simulink model "sampleModel7127_pp_difftest"  (R2018a)
settings: Solver=VariableStepAuto  StartTime=0.0  StopTime=10.0  RelTol=1e-3
undefined symbols (not defined in the file or in its folder): DiscIntNeverNeededParam, sigbuilder_block
libraries: simulink x258
(part 1 of 5)
settings Model: Creator=cyfuzz  LastModifiedBy=ishaf
settings CodeAppCC: StateflowObjectComments=on

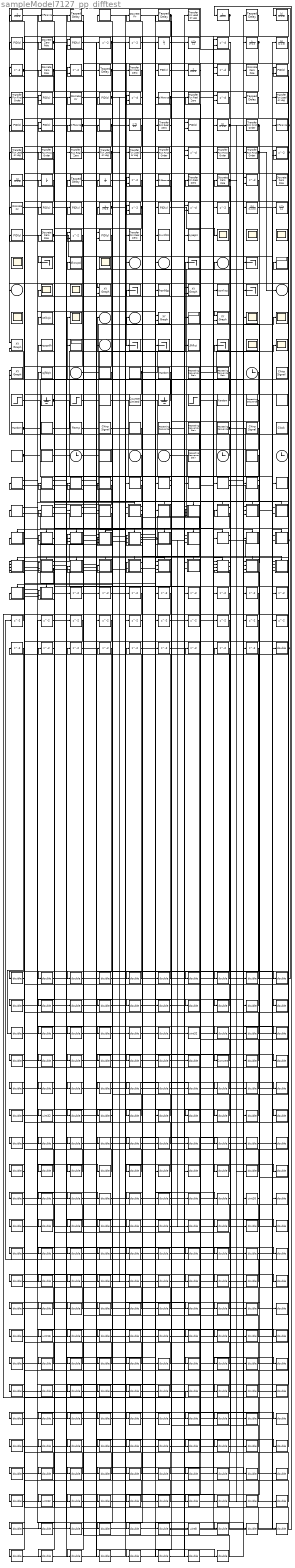
== system sampleModel7127_pp_difftest ==
  cfblk133 : Inport
  cfblk165 : Inport  Port=2
  cfblk166 : Inport  Port=3
  cfblk{1,8,19,27,74} (5 alike) : DiscreteTransferFcn  SampleTime=1
  cfblk{10,20,48,61,79} (5 alike) : DiscreteFilter  SampleTime=1
  cfblk100 : Display
  cfblk{88..91,94,102..103,111,113,119..120,129..130} (13 alike) : Scope
      cfblk103 settings: Floating=on
      cfblk111 settings: Floating=on
      cfblk129 settings: Floating=on
      cfblk89 settings: Floating=on
      cfblk90 settings: Floating=on
      cfblk91 settings: Floating=on
      cfblk94 settings: Floating=on
  cfblk{104,107,116,118,121,131} (6 alike) : simulink/Sinks/XY Graph  xmin=-1  xmax=1  ymin=-1  ymax=1  st=-1
  cfblk{92,97,99,105,109,125..126,128} (8 alike) : Terminator
  cfblk106 : ToWorkspace  VariableName=hqnbljg  SaveFormat=Timeseries  SampleTime=-1
  cfblk108 : ToWorkspace  VariableName=kqrxkcy  SaveFormat=Timeseries  SampleTime=-1
  cfblk{11,26,34,41,72..73,76,81} (8 alike) : simulink/Continuous/PID Controller  Controller=PID  TimeDomain=Discrete-time  SampleTime=1  IntegratorMethod=Forward Euler  FilterMethod=Forward Euler  Form=Parallel  UseFilter=on  ControllerParametersSource=internal  P=1  I=1  D=0  N=100  InitialConditionSource=internal  InitialConditionForIntegrator=0  InitialConditionForFilter=0  ExternalReset=none  LimitOutput=off  UpperSaturationLimit=inf  LowerSaturationLimit=-inf  LinearizeAsGain=off  AntiWindupMode=none  Kb=1  TrackingMode=off  Kt=1  PParamMin=[]  PParamMax=[]  IParamMin=[]  IParamMax=[]  DParamMin=[]  DParamMax=[]  NParamMin=[]  NParamMax=[]  KbParamMin=[]  KbParamMax=[]  KtParamMin=[]  KtParamMax=[]  POutMin=[]  POutMax=[]  IOutMin=[]  IOutMax=[]  DOutMin=[]  DOutMax=[]  NOutMin=[]  NOutMax=[]  KbOutMin=[]  KbOutMax=[]  KtOutMin=[]  KtOutMax=[]  IntegratorOutMin=[]  IntegratorOutMax=[]  FilterOutMin=[]  FilterOutMax=[]  SumOutMin=[]  SumOutMax=[]  SumI1OutMin=[]  SumI1OutMax=[]  SumI2OutMin=[]  SumI2OutMax=[]  SumI3OutMin=[]  SumI3OutMax=[]  SumDOutMin=[]  SumDOutMax=[]  SaturationOutMin=[]  SaturationOutMax=[]  IntegratorContinuousStateAttributes=''  IntegratorStateMustResolveToSignalObject=off  IntegratorRTWStateStorageClass=Auto  FilterContinuousStateAttributes=''  FilterStateMustResolveToSignalObject=off  FilterRTWStateStorageClass=Auto  DifferentiatorICPrevScaledInput=0  DifferentiatorOutMin=[]  DifferentiatorOutMax=[]  FilterDiffOutCoefMin=[]  FilterDiffOutCoefMax=[]  SumDenOutMin=[]  SumDenOutMax=[]  SumNumOutMin=[]  SumNumOutMax=[]  ReciprocalOutMin=[]  ReciprocalOutMax=[]  DivideOutMin=[]  DivideOutMax=[]  TunerSelectOption=Transfer Function Based (PID Tuner App)
  cfblk112 : ToWorkspace  VariableName=otikzjx  SaveFormat=Timeseries  SampleTime=-1
  cfblk117 : Display
  cfblk{12,22,29,68,70,82} (6 alike) : DiscreteZeroPole  Poles=[0 0.5]  Gain=1
  cfblk122 : ToWorkspace  VariableName=rqzqsdh  SaveFormat=Timeseries  SampleTime=-1
  cfblk123 : Display
  cfblk127 : ToWorkspace  VariableName=jlhlkzi  SaveFormat=Timeseries  SampleTime=-1
  cfblk{13,30,32,42,47,84} (6 alike) : simulink/Continuous/PID Controller (2DOF)  Controller=PID  TimeDomain=Discrete-time  SampleTime=1  IntegratorMethod=Forward Euler  FilterMethod=Forward Euler  Form=Parallel  UseFilter=on  ControllerParametersSource=internal  P=1  I=1  D=0  N=100  b=1  c=1  InitialConditionSource=internal  InitialConditionForIntegrator=0  InitialConditionForFilter=0  ExternalReset=none  LimitOutput=off  UpperSaturationLimit=inf  LowerSaturationLimit=-inf  LinearizeAsGain=off  AntiWindupMode=none  Kb=1  TrackingMode=off  Kt=1  PParamMin=[]  PParamMax=[]  IParamMin=[]  IParamMax=[]  DParamMin=[]  DParamMax=[]  NParamMin=[]  NParamMax=[]  bParamMin=[]  bParamMax=[]  cParamMin=[]  cParamMax=[]  KbParamMin=[]  KbParamMax=[]  KtParamMin=[]  KtParamMax=[]  POutMin=[]  POutMax=[]  IOutMin=[]  IOutMax=[]  DOutMin=[]  DOutMax=[]  NOutMin=[]  NOutMax=[]  bOutMin=[]  bOutMax=[]  cOutMin=[]  cOutMax=[]  KbOutMin=[]  KbOutMax=[]  KtOutMin=[]  KtOutMax=[]  IntegratorOutMin=[]  IntegratorOutMax=[]  FilterOutMin=[]  FilterOutMax=[]  SumOutMin=[]  SumOutMax=[]  Sum1OutMin=[]  Sum1OutMax=[]  Sum2OutMin=[]  Sum2OutMax=[]  Sum3OutMin=[]  Sum3OutMax=[]  SumI1OutMin=[]  SumI1OutMax=[]  SumI2OutMin=[]  SumI2OutMax=[]  SumI3OutMin=[]  SumI3OutMax=[]  SumDOutMin=[]  SumDOutMax=[]  SaturationOutMin=[]  SaturationOutMax=[]  IntegratorContinuousStateAttributes=''  IntegratorStateMustResolveToSignalObject=off  IntegratorRTWStateStorageClass=Auto  FilterContinuousStateAttributes=''  FilterStateMustResolveToSignalObject=off  FilterRTWStateStorageClass=Auto  DifferentiatorICPrevScaledInput=0  DifferentiatorOutMin=[]  DifferentiatorOutMax=[]  FilterDiffOutCoefMin=[]  FilterDiffOutCoefMax=[]  SumDenOutMin=[]  SumDenOutMax=[]  SumNumOutMin=[]  SumNumOutMax=[]  ReciprocalOutMin=[]  ReciprocalOutMax=[]  DivideOutMin=[]  DivideOutMax=[]  TunerSelectOption=Transfer Function Based (PID Tuner App)
  cfblk132 : ToWorkspace  VariableName=qjfdqit  SaveFormat=Timeseries  SampleTime=-1
  cfblk{134..135,161,169} (4 alike) : simulink/Sources/Band-Limited White Noise  Cov=[0.1]  Ts=0.1  seed=[23341]
  cfblk136 : RandomNumber  SampleTime=0.1
  cfblk{137..138,157,167} (4 alike) : simulink/Sources/Repeating Sequence Stair  OutValues=[3 1 4 2 1].'  tsamp=1  OutMin=[]  OutMax=[]  OutDataTypeStr=double  OutputDataTypeScalingMode=double  OutDataType=fixdt(0,8)  ConRadixGroup=Best Precision: Vector-wise  OutScaling=2^-12
  cfblk{139,163,168,170} (4 alike) : Clock
  cfblk{14..15,78,213..239} (30 alike) : Delay  SampleTime=1
  cfblk140 : simulink/Sources/Chirp Signal  f1=0.1  T=100  f2=1
  cfblk141 : Step  After=53  SampleTime=0
  cfblk142 : Ground
  cfblk143 : Step  After=78  SampleTime=0
  cfblk144 : simulink/Sources/Counter Free-Running  NumBits=16  tsamp=1
  cfblk145 : simulink/Sources/Counter Limited  uplimit=7  tsamp=1
  cfblk146 : Ground
  cfblk147 : Step  After=42  SampleTime=0
  cfblk148 : RandomNumber  SampleTime=0.1
  cfblk149 : simulink/Sources/Repeating Sequence  rep_seq_t=[0 2]  rep_seq_y=[0 2]
  cfblk150 : simulink/Sources/Repeating Sequence Interpolated  OutValues=[3 1 4 2 1].'  TimeValues=[0 0.1 0.5 0.6 1].'  LookUpMeth=Interpolation-Use End Values  tsamp=0.01  OutMin=[]  OutMax=[]  OutDataTypeStr=double  OutputDataTypeScalingMode=double  OutDataType=fixdt(0,8)  OutScaling=2^-10
  cfblk151 : UniformRandomNumber  SampleTime=0.1
  cfblk152 : simulink/Sources/Repeating Sequence Interpolated  OutValues=[3 1 4 2 1].'  TimeValues=[0 0.1 0.5 0.6 1].'  LookUpMeth=Interpolation-Use End Values  tsamp=0.01  OutMin=[]  OutMax=[]  OutDataTypeStr=double  OutputDataTypeScalingMode=double  OutDataType=fixdt(0,8)  OutScaling=2^-10
  cfblk153 : simulink/Sources/Ramp  slope=1  start=0  InitialOutput=0
  cfblk154 : simulink/Sources/Chirp Signal  f1=0.1  T=100  f2=1
  cfblk155 : simulink/Sources/Counter Free-Running  NumBits=16  tsamp=1
  cfblk156 : simulink/Sources/Repeating Sequence  rep_seq_t=[0 2]  rep_seq_y=[0 2]
  cfblk158 : simulink/Sources/Repeating Sequence  rep_seq_t=[0 2]  rep_seq_y=[0 2]
  cfblk159 : simulink/Sources/Chirp Signal  f1=0.1  T=100  f2=1
  cfblk16 : UnitDelay
  cfblk160 : DigitalClock
  cfblk162 : Subsystem  Tag=STV Subsys  LoadFcn=sigbuilder_block('load');  StartFcn=sigbuilder_block('start');  StopFcn=sigbuilder_block('stop');  ClipboardFcn=sigbuilder_block('clipboard');  mask(Sigbuilder block){tuvar=[0:10]}
      mask help: Simulink:masks:SigbuilderBlock_MD
      mask init:
      | if ~strcmp(get_param(bdroot(gcbh),'SimulationStatus'),'stopped') tuvar = sigbuilder_block('maskInit'); end
      settings: CopyFcn=sigbuilder_block('copy');  DeleteFcn=sigbuilder_block('delete');  ModelCloseFcn=sigbuilder_block('modelClose');  PreSaveFcn=sigbuilder_block('preSave');  PauseFcn=sigbuilder_block('pause');  ContinueFcn=sigbuilder_block('continue');  NameChangeFcn=sigbuilder_block('namechange');  OpenFcn=sigbuilder_block('open',[437.6 199.2 550.4 400 ]);  CloseFcn=sigbuilder_block('close');
      mask Display: plot(0, 0, 100, 100,[2, 2, 32, 32, 2], [68, 8, 8, 68, 68],[32, 2], [38, 38], [32, 19, 2],[53, 60, 44], [32, 17, 17, 2],[16, 16, 31, 31]);txt = getActiveGroup(gcbh);text(2, 100, txt,'verticalAlignment', 'top');
  cfblk164 : Subsystem  Tag=STV Subsys  LoadFcn=sigbuilder_block('load');  StartFcn=sigbuilder_block('start');  StopFcn=sigbuilder_block('stop');  ClipboardFcn=sigbuilder_block('clipboard');  mask(Sigbuilder block){tuvar=[0:10]}
      mask help: Simulink:masks:SigbuilderBlock_MD
      mask init:
      | if ~strcmp(get_param(bdroot(gcbh),'SimulationStatus'),'stopped') tuvar = sigbuilder_block('maskInit'); end
      settings: CopyFcn=sigbuilder_block('copy');  DeleteFcn=sigbuilder_block('delete');  ModelCloseFcn=sigbuilder_block('modelClose');  PreSaveFcn=sigbuilder_block('preSave');  PauseFcn=sigbuilder_block('pause');  ContinueFcn=sigbuilder_block('continue');  NameChangeFcn=sigbuilder_block('namechange');  OpenFcn=sigbuilder_block('open',[437.6 199.2 550.4 400 ]);  CloseFcn=sigbuilder_block('close');
      mask Display: plot(0, 0, 100, 100,[2, 2, 32, 32, 2], [68, 8, 8, 68, 68],[32, 2], [38, 38], [32, 19, 2],[53, 60, 44], [32, 17, 17, 2],[16, 16, 31, 31]);txt = getActiveGroup(gcbh);text(2, 100, txt,'verticalAlignment', 'top');
  cfblk17 : DiscreteIntegrator  OutDataTypeStr=double  ICPrevOutput=DiscIntNeverNeededParam  ICPrevScaledInput=DiscIntNeverNeededParam
  cfblk{171..184} (14 alike) : If  SampleTime=1
  cfblk{18,28,35,38,57,69,77} (7 alike) : Delay  DelayLengthSource=Input port  SampleTime=1
      settings: InputPortMap=u0,p1
  cfblk185 : Subsystem  TreatAsAtomicUnit=on
  cfblk186 : Subsystem  TreatAsAtomicUnit=on
  cfblk187 : Subsystem  TreatAsAtomicUnit=on
  cfblk188 : Subsystem  TreatAsAtomicUnit=on
  cfblk189 : Subsystem  TreatAsAtomicUnit=on
  cfblk190 : Subsystem  TreatAsAtomicUnit=on
  cfblk191 : Subsystem  TreatAsAtomicUnit=on
  cfblk192 : Subsystem  TreatAsAtomicUnit=on
  cfblk193 : Subsystem  TreatAsAtomicUnit=on
  cfblk194 : Subsystem  TreatAsAtomicUnit=on
  cfblk195 : Subsystem  TreatAsAtomicUnit=on
  cfblk196 : Subsystem  TreatAsAtomicUnit=on
  cfblk197 : Subsystem  TreatAsAtomicUnit=on
  cfblk198 : Subsystem  TreatAsAtomicUnit=on
  cfblk199 : Subsystem  TreatAsAtomicUnit=on
  cfblk{2,36,43,50,66} (5 alike) : simulink/Discrete/Difference  ICPrevInput=0.0  OutMin=[]  OutMax=[]  OutDataTypeStr=double  OutputDataTypeScalingMode=double  OutDataType=fixdt(1, 16)  OutScaling=2^-10  DoSatur=off
  cfblk200 : Subsystem  TreatAsAtomicUnit=on
  cfblk201 : Subsystem  TreatAsAtomicUnit=on
  cfblk202 : Subsystem  TreatAsAtomicUnit=on
  cfblk203 : Subsystem  TreatAsAtomicUnit=on
  cfblk204 : Subsystem  TreatAsAtomicUnit=on
  cfblk205 : Subsystem  TreatAsAtomicUnit=on
  cfblk206 : Subsystem  TreatAsAtomicUnit=on
  cfblk207 : Subsystem  TreatAsAtomicUnit=on
  cfblk208 : Subsystem  TreatAsAtomicUnit=on
  cfblk209 : Subsystem  TreatAsAtomicUnit=on
  cfblk{21,23,60,65,75,83} (6 alike) : Delay  ShowEnablePort=on  SampleTime=1
      settings: InputPortMap=u0,e6
  cfblk210 : Subsystem  TreatAsAtomicUnit=on
  cfblk211 : Subsystem  TreatAsAtomicUnit=on
  cfblk212 : Subsystem  TreatAsAtomicUnit=on
  cfblk{3,6,9,24,39,63} (6 alike) : simulink/Discrete/Tapped Delay  vinit=0.0  samptime=-1  NumDelays=1  DelayOrder=Oldest  includeCurrent=off
  cfblk240 : DataTypeConversion  OutDataTypeStr=double
  cfblk{25,37,46,53,67,85} (6 alike) : simulink/Discrete/Transfer Fcn Real Zero  ZeroZ=0.75  ICPrevInput=0.0  DoSatur=off
      settings: SourceProductName=Simulink  SourceProductBaseCode=SL
  cfblk{31,49,52,56,58..59} (6 alike) : simulink/Discrete/Transfer Fcn First Order  PoleZ=0.95  ICPrevOutput=0.0  DoSatur=off
      settings: SourceProductName=Simulink
  cfblk33 : DiscreteFir  SampleTime=1
  cfblk4 : DiscreteStateSpace
  cfblk{7,40,51,54..55} (5 alike) : simulink/Discrete/Transfer Fcn Lead or Lag  PoleZ=0.95  ZeroZ=0.75  ICPrevOutput=0.0  ICPrevInput=0.0  DoSatur=off
      settings: SourceProductName=Simulink  SourceProductBaseCode=SL
  cfblk44 : DiscreteStateSpace
  cfblk45 : DiscreteIntegrator  OutDataTypeStr=double  ICPrevOutput=DiscIntNeverNeededParam  ICPrevScaledInput=DiscIntNeverNeededParam
  cfblk5 : DiscreteFir  SampleTime=1
  cfblk62 : UnitDelay
  cfblk64 : UnitDelay
  cfblk71 : DiscreteFir  SampleTime=1
  cfblk80 : DiscreteIntegrator  OutDataTypeStr=uint8  ICPrevOutput=DiscIntNeverNeededParam  ICPrevScaledInput=DiscIntNeverNeededParam
  cfblk86 : ToWorkspace  VariableName=zvvzltm  SaveFormat=Timeseries  SampleTime=-1
  cfblk87 : ToWorkspace  VariableName=sypegzn  SaveFormat=Timeseries  SampleTime=-1
  cfblk93 : ToWorkspace  VariableName=dkovpci  SaveFormat=Timeseries  SampleTime=-1
  cyemi_{0..25,27..33,69,185..186,188,204,213..215,220..222,256,270..271,279..280,299..302,329..331,371,382..384,425,435,446..449,455..458,519..520,530,544,554..555,563..565,587..588,623..626,693..694,705..710,728,766..767,776..806,808..866,868..881,883..893} (211 alike) : DataTypeConversion  OutDataTypeStr=double
  cyemi_187 : DataTypeConversion  OutDataTypeStr=fixdt('ufix64_En32')
  cyemi_26 : DataTypeConversion  OutDataTypeStr=uint32
  cyemi_281 : DataTypeConversion  OutDataTypeStr=uint32
  cyemi_692 : DataTypeConversion  OutDataTypeStr=uint16
  cyemi_807 : DataTypeConversion  OutDataTypeStr=uint16
  cyemi_867 : DataTypeConversion  OutDataTypeStr=uint32
  cyemi_882 : DataTypeConversion  OutDataTypeStr=uint8
  cfblk95 : Outport
  cfblk96 : Outport  Port=2
  cfblk98 : Outport  Port=3
  cfblk101 : Outport  Port=4
  cfblk110 : Outport  Port=5
  cfblk114 : Outport  Port=6
  cfblk115 : Outport  Port=7
  cfblk124 : Outport  Port=8
  wires:
  cfblk17/1 -> cfblk125/1, cyemi_839/1
  cfblk49/1 -> cyemi_804/1, cyemi_858/1
  cfblk28/1 -> cfblk121/1
  cfblk148/1 -> cfblk113/1
  cfblk50/1 -> cfblk118/1, cyemi_707/1
  cfblk64/1 -> cfblk95/1
  cfblk6/1 -> cyemi_0/1, cyemi_709/1
  cfblk202/1(cfblk2) -> cfblk120/1
  cfblk72/1 -> cfblk126/1
  cfblk167/1 -> cfblk131/1
  cfblk201/1(cfblk2) -> cfblk123/1
  cfblk24/1 -> cyemi_449/1, cyemi_838/1
  cfblk142/1 -> cyemi_3/1, cyemi_889/1
  cfblk195/2(cfblk15) -> cfblk98/1
  cfblk133/1 -> cfblk97/1
  cfblk36/1 -> cyemi_9/1, cyemi_435/1
  cfblk160/1 -> cfblk100/1
  cfblk209/1(cfblk2) -> cfblk119/1
  cfblk68/1 -> cyemi_8/1, cyemi_811/1, cyemi_819/1, cyemi_874/1
  cfblk199/2(cfblk10) -> cfblk128/1
  cfblk195/4(cfblk17) -> cfblk105/1
  cfblk1/1 -> cfblk116/1
  cfblk54/1 -> cyemi_24/1, cyemi_886/1
  cfblk135/1 -> cfblk107/2, cyemi_846/1
  cfblk82/1 -> cyemi_784/1, cyemi_885/1
  cfblk22/1 -> cyemi_14/1, cyemi_30/1
  cfblk21/1 -> cyemi_780/1, cyemi_843/1
  cfblk75/1 -> cfblk92/1, cyemi_887/1
  cfblk197/1(cfblk2) -> cfblk115/1
  cfblk161/1 -> cfblk109/1, cyemi_878/1
  cfblk151/1 -> cyemi_447/1, cyemi_810/1
  cfblk152/1 -> cfblk114/1
  cfblk48/1 -> cyemi_555/1, cyemi_803/1, cyemi_825/1
  cfblk47/1 -> cyemi_23/1, cyemi_694/1
  cfblk74/1 -> cyemi_33/1, cyemi_785/1
  cfblk34/1 -> cyemi_790/1, cyemi_791/1
  cfblk12/1 -> cyemi_11/1, cyemi_330/1
  cfblk158/1 -> cyemi_693/1, cyemi_823/1
  cfblk80/1 -> cfblk101/1
  cfblk43/1 -> cyemi_708/1, cyemi_893/1
  cfblk137/1 -> cfblk130/1, cyemi_15/1, cyemi_302/1
  cfblk168/1 -> cfblk96/1
  cfblk207/3(cfblk16) -> cfblk124/1
  cfblk202/3(cfblk13) -> cyemi_800/1, cyemi_866/1
  cfblk44/1 -> cyemi_299/1, cyemi_802/1
  cfblk77/1 -> cfblk104/1
  cfblk197/3(cfblk16) -> cfblk102/1
  cfblk150/1 -> cfblk116/2
  cfblk193/2(cfblk17) -> cfblk104/2
  cfblk146/1 -> cfblk121/2
  cfblk205/2(cfblk9) -> cfblk117/1
  cfblk134/1 -> cfblk131/2
  cfblk14/1 -> cyemi_706/1, cyemi_873/1, cyemi_888/1
  cfblk19/1 -> cyemi_798/1, cyemi_862/1
  cfblk60/1 -> cyemi_371/1, cyemi_808/1
  cfblk59/1 -> cfblk110/1, cyemi_21/1
  cfblk200/2(cfblk8) -> cyemi_796/1, cyemi_868/1
  cfblk76/1 -> cfblk88/1
  cfblk196/2(cfblk10) -> cyemi_710/1, cyemi_864/1
  cfblk204/3(cfblk10) -> cyemi_271/1, cyemi_812/1
  cfblk170/1 -> cfblk107/1
  cfblk8/1 -> cfblk118/2, cyemi_797/1
  cfblk203/3(cfblk9) -> cfblk99/1
  cfblk171/1 -> cfblk185/Action
  cfblk171/2 -> cfblk186/Action
  cfblk172/1 -> cfblk187/Action
  cfblk172/2 -> cfblk188/Action
  cfblk173/1 -> cfblk189/Action
  cfblk173/2 -> cfblk190/Action
  cfblk174/1 -> cfblk191/Action
  cfblk174/2 -> cfblk192/Action
  cfblk175/1 -> cfblk193/Action
  cfblk175/2 -> cfblk194/Action
  cfblk176/1 -> cfblk195/Action
  cfblk176/2 -> cfblk196/Action
  cfblk177/1 -> cfblk197/Action
  cfblk177/2 -> cfblk198/Action
  cfblk178/1 -> cfblk199/Action
  cfblk178/2 -> cfblk200/Action
  cfblk179/1 -> cfblk201/Action
  cfblk179/2 -> cfblk202/Action
  cfblk180/1 -> cfblk203/Action
  cfblk180/2 -> cfblk204/Action
  cfblk181/1 -> cfblk205/Action
  cfblk181/2 -> cfblk206/Action
  cfblk182/1 -> cfblk207/Action
  cfblk182/2 -> cfblk208/Action
  cfblk183/1 -> cfblk209/Action
  cfblk183/2 -> cfblk210/Action
  cfblk184/1 -> cfblk211/Action
  cfblk184/2 -> cfblk212/Action
  cfblk240/1 -> cyemi_783/1, cyemi_871/1
  cyemi_0/1 -> cfblk1/1
  cyemi_1/1 -> cfblk10/1
  cfblk138/1 -> cyemi_1/1
  cyemi_2/1 -> cfblk106/1
  cfblk207/2(cfblk15) -> cyemi_2/1
  cyemi_3/1 -> cfblk108/1
  cyemi_4/1 -> cfblk11/1
  cfblk205/1(cfblk2) -> cyemi_4/1
  cyemi_5/1 -> cfblk112/1
  cfblk46/1 -> cyemi_5/1
  cyemi_6/1 -> cfblk12/1
  cfblk27/1 -> cyemi_6/1
  cyemi_7/1 -> cfblk122/1
  cfblk63/1 -> cyemi_7/1
  cyemi_8/1 -> cfblk127/1
  cyemi_9/1 -> cfblk13/1
  cyemi_10/1 -> cfblk13/2
  cfblk39/1 -> cyemi_10/1
  cyemi_11/1 -> cfblk132/1
  cyemi_12/1 -> cfblk14/1
  cfblk212/1(cfblk2) -> cyemi_12/1
  cyemi_13/1 -> cfblk15/1
  cfblk164/1(Signal 1) -> cyemi_13/1
  cyemi_14/1 -> cfblk16/1
  cyemi_15/1 -> cfblk17/1
  cyemi_16/1 -> cfblk171/1
  cfblk51/1 -> cyemi_16/1
  cyemi_17/1 -> cfblk172/1
  cfblk18/1 -> cyemi_17/1
  cyemi_18/1 -> cfblk173/1
  cfblk16/1 -> cyemi_18/1
  cyemi_19/1 -> cfblk174/1
  cfblk30/1 -> cyemi_19/1
  cyemi_20/1 -> cfblk175/1
  cfblk231/1 -> cyemi_20/1
  cyemi_21/1 -> cfblk176/1
  cyemi_22/1 -> cfblk177/1
  cfblk45/1 -> cyemi_22/1
  cyemi_23/1 -> cfblk178/1
  cyemi_24/1 -> cfblk179/1
  cyemi_25/1 -> cfblk18/1
  cfblk31/1 -> cyemi_25/1
  cyemi_26/1 -> cfblk18/2
  cfblk203/4(cfblk10) -> cyemi_26/1
  cyemi_27/1 -> cfblk180/1
  cfblk211/2(cfblk14) -> cyemi_27/1
  cyemi_28/1 -> cfblk181/1
  cfblk190/1(cfblk2) -> cyemi_28/1
  cyemi_29/1 -> cfblk182/1
  cfblk41/1 -> cyemi_29/1
  cyemi_30/1 -> cfblk183/1
  cyemi_31/1 -> cfblk184/1
  cfblk238/1 -> cyemi_31/1
  cyemi_32/1 -> cfblk185/1(cfblk1)
  cfblk186/1(cfblk2) -> cyemi_32/1
  cyemi_33/1 -> cfblk185/2(cfblk14)
  cyemi_69/1 -> cfblk186/1(cfblk1)
  cfblk20/1 -> cyemi_69/1
  cyemi_185/1 -> cfblk187/1(cfblk1)
  cfblk208/1(cfblk2) -> cyemi_185/1
  cyemi_186/1 -> cfblk187/2(cfblk13)
  cfblk226/1 -> cyemi_186/1
  cyemi_187/1 -> cfblk187/3(cfblk14)
  cfblk203/2(cfblk8) -> cyemi_187/1
  cyemi_188/1 -> cfblk187/4(cfblk15)
  cfblk236/1 -> cyemi_188/1
  cyemi_204/1 -> cfblk188/1(cfblk1)
  cfblk214/1 -> cyemi_204/1
  cyemi_213/1 -> cfblk189/1(cfblk1)
  cfblk219/1 -> cyemi_213/1
  cyemi_214/1 -> cfblk189/2(cfblk7)
  cfblk224/1 -> cyemi_214/1
  cyemi_215/1 -> cfblk189/3(cfblk8)
  cfblk229/1 -> cyemi_215/1
  cyemi_220/1 -> cfblk19/1
  cfblk9/1 -> cyemi_220/1
  cyemi_221/1 -> cfblk190/1(cfblk1)
  cfblk197/2(cfblk15) -> cyemi_221/1
  cyemi_222/1 -> cfblk190/2(cfblk13)
  cfblk56/1 -> cyemi_222/1
  cyemi_256/1 -> cfblk191/1(cfblk1)
  cfblk156/1 -> cyemi_256/1
  cyemi_270/1 -> cfblk192/1(cfblk1)
  cfblk53/1 -> cyemi_270/1
  cyemi_271/1 -> cfblk192/2(cfblk8)
  cyemi_279/1 -> cfblk193/1(cfblk1)
  cfblk13/1 -> cyemi_279/1
  cyemi_280/1 -> cfblk193/2(cfblk15)
  cfblk223/1 -> cyemi_280/1
  cyemi_281/1 -> cfblk193/3(cfblk16)
  cfblk203/1(cfblk2) -> cyemi_281/1
  cyemi_299/1 -> cfblk194/1(cfblk1)
  cyemi_300/1 -> cfblk194/2(cfblk6)
  cfblk230/1 -> cyemi_300/1
  cyemi_301/1 -> cfblk194/3(cfblk7)
  cfblk208/3(cfblk17) -> cyemi_301/1
  cyemi_302/1 -> cfblk194/4(cfblk8)
  cyemi_329/1 -> cfblk195/1(cfblk1)
  cfblk237/1 -> cyemi_329/1
  cyemi_330/1 -> cfblk195/2(cfblk13)
  cyemi_331/1 -> cfblk195/3(cfblk14)
  cfblk227/1 -> cyemi_331/1
  cyemi_371/1 -> cfblk196/1(cfblk1)
  cyemi_382/1 -> cfblk197/1(cfblk1)
  cfblk62/1 -> cyemi_382/1
  cyemi_383/1 -> cfblk197/2(cfblk13)
  cfblk232/1 -> cyemi_383/1
  cyemi_384/1 -> cfblk197/3(cfblk14)
  cfblk73/1 -> cyemi_384/1
  cyemi_425/1 -> cfblk198/1(cfblk1)
  cfblk208/2(cfblk16) -> cyemi_425/1
  cyemi_435/1 -> cfblk199/1(cfblk1)
  cyemi_446/1 -> cfblk2/1
  cfblk228/1 -> cyemi_446/1
  cyemi_447/1 -> cfblk20/1
  cyemi_448/1 -> cfblk200/1(cfblk1)
  cfblk70/1 -> cyemi_448/1
  cyemi_449/1 -> cfblk200/2(cfblk7)
  cyemi_455/1 -> cfblk201/1(cfblk1)
  cfblk153/1 -> cyemi_455/1
  cyemi_456/1 -> cfblk201/2(cfblk8)
  cfblk239/1 -> cyemi_456/1
  cyemi_457/1 -> cfblk201/3(cfblk9)
  cfblk218/1 -> cyemi_457/1
  cyemi_458/1 -> cfblk201/4(cfblk10)
  cfblk234/1 -> cyemi_458/1
  cyemi_519/1 -> cfblk202/1(cfblk1)
  cfblk61/1 -> cyemi_519/1
  cyemi_520/1 -> cfblk202/2(cfblk11)
  cfblk225/1 -> cyemi_520/1
  cyemi_530/1 -> cfblk203/1(cfblk1)
  cfblk162/1(Signal 1) -> cyemi_530/1
  cyemi_544/1 -> cfblk204/1(cfblk1)
  cfblk154/1 -> cyemi_544/1
  cyemi_554/1 -> cfblk205/1(cfblk1)
  cfblk4/1 -> cyemi_554/1
  cyemi_555/1 -> cfblk205/2(cfblk8)
  cyemi_563/1 -> cfblk206/1(cfblk1)
  cfblk15/1 -> cyemi_563/1
  cyemi_564/1 -> cfblk206/2(cfblk16)
  cfblk215/1 -> cyemi_564/1
  cyemi_565/1 -> cfblk206/3(cfblk17)
  cfblk217/1 -> cyemi_565/1
  cyemi_587/1 -> cfblk207/1(cfblk1)
  cfblk191/1(cfblk2) -> cyemi_587/1
  cyemi_588/1 -> cfblk207/2(cfblk14)
  cfblk222/1 -> cyemi_588/1
  cyemi_623/1 -> cfblk208/1(cfblk1)
  cfblk216/1 -> cyemi_623/1
  cyemi_624/1 -> cfblk208/2(cfblk13)
  cfblk149/1 -> cyemi_624/1
  cyemi_625/1 -> cfblk208/3(cfblk14)
  cfblk141/1 -> cyemi_625/1
  cyemi_626/1 -> cfblk208/4(cfblk15)
  cfblk235/1 -> cyemi_626/1
  cyemi_692/1 -> cfblk209/1(cfblk1)
  cfblk144/1 -> cyemi_692/1
  cyemi_693/1 -> cfblk209/2(cfblk12)
  cyemi_694/1 -> cfblk209/3(cfblk13)
  cyemi_705/1 -> cfblk21/1
  cfblk206/1(cfblk2) -> cyemi_705/1
  cyemi_706/1 -> cfblk21/2
  cyemi_707/1 -> cfblk210/1(cfblk1)
  cyemi_708/1 -> cfblk210/2(cfblk15)
  cyemi_709/1 -> cfblk210/3(cfblk16)
  cyemi_710/1 -> cfblk210/4(cfblk17)
  cyemi_728/1 -> cfblk211/1(cfblk1)
  cfblk2/1 -> cyemi_728/1
  cyemi_766/1 -> cfblk212/1(cfblk1)
  cfblk220/1 -> cyemi_766/1
  cyemi_767/1 -> cfblk212/2(cfblk9)
  cfblk233/1 -> cyemi_767/1
  cyemi_776/1 -> cfblk213/1
  cfblk201/2(cfblk11) -> cyemi_776/1
  cyemi_777/1 -> cfblk214/1
  cfblk84/1 -> cyemi_777/1
  cyemi_778/1 -> cfblk215/1
  cfblk188/1(cfblk2) -> cyemi_778/1
  cyemi_779/1 -> cfblk216/1
  cfblk32/1 -> cyemi_779/1
  cyemi_780/1 -> cfblk217/1
  cyemi_781/1 -> cfblk218/1
  cfblk188/2(cfblk11) -> cyemi_781/1
  cyemi_782/1 -> cfblk219/1
  cfblk42/1 -> cyemi_782/1
  cyemi_783/1 -> cfblk22/1
  cyemi_784/1 -> cfblk220/1
  cyemi_785/1 -> cfblk221/1
  cyemi_786/1 -> cfblk222/1
  cfblk185/1(cfblk2) -> cyemi_786/1
  cyemi_787/1 -> cfblk223/1
  cfblk185/2(cfblk15) -> cyemi_787/1
  cyemi_788/1 -> cfblk224/1
  cfblk3/1 -> cyemi_788/1
  cyemi_789/1 -> cfblk225/1
  cfblk185/3(cfblk16) -> cyemi_789/1
  cyemi_790/1 -> cfblk226/1
  cyemi_791/1 -> cfblk227/1
  cyemi_792/1 -> cfblk228/1
  cfblk23/1 -> cyemi_792/1
  cyemi_793/1 -> cfblk229/1
  cfblk26/1 -> cyemi_793/1
  cyemi_794/1 -> cfblk23/1
  cfblk5/1 -> cyemi_794/1
  cyemi_795/1 -> cfblk23/2
  cfblk211/3(cfblk15) -> cyemi_795/1
  cyemi_796/1 -> cfblk230/1
  cyemi_797/1 -> cfblk231/1
  cyemi_798/1 -> cfblk232/1
  cyemi_799/1 -> cfblk233/1
  cfblk65/1 -> cyemi_799/1
  cyemi_800/1 -> cfblk234/1
  cyemi_801/1 -> cfblk235/1
  cfblk194/2(cfblk9) -> cyemi_801/1
  cyemi_802/1 -> cfblk236/1
  cyemi_803/1 -> cfblk237/1
  cyemi_804/1 -> cfblk238/1
  cyemi_805/1 -> cfblk239/1
  cfblk198/2(cfblk10) -> cyemi_805/1
  cyemi_806/1 -> cfblk24/1
  cfblk52/1 -> cyemi_806/1
  cyemi_807/1 -> cfblk240/1
  cfblk155/1 -> cyemi_807/1
  cyemi_808/1 -> cfblk25/1
  cyemi_809/1 -> cfblk26/1
  cfblk200/1(cfblk2) -> cyemi_809/1
  cyemi_810/1 -> cfblk27/1
  cyemi_811/1 -> cfblk28/1
  cyemi_812/1 -> cfblk28/2
  cyemi_813/1 -> cfblk29/1
  cfblk211/1(cfblk2) -> cyemi_813/1
  cyemi_814/1 -> cfblk3/1
  cfblk193/1(cfblk2) -> cyemi_814/1
  cyemi_815/1 -> cfblk30/1
  cfblk71/1 -> cyemi_815/1
  cyemi_816/1 -> cfblk30/2
  cfblk66/1 -> cyemi_816/1
  cyemi_817/1 -> cfblk31/1
  cfblk165/1 -> cyemi_817/1
  cyemi_818/1 -> cfblk32/1
  cfblk210/1(cfblk2) -> cyemi_818/1
  cyemi_819/1 -> cfblk32/2
  cyemi_820/1 -> cfblk33/1
  cfblk10/1 -> cyemi_820/1
  cyemi_821/1 -> cfblk34/1
  cfblk202/2(cfblk12) -> cyemi_821/1
  cyemi_822/1 -> cfblk35/1
  cfblk38/1 -> cyemi_822/1
  cyemi_823/1 -> cfblk35/2
  cyemi_824/1 -> cfblk36/1
  cfblk37/1 -> cyemi_824/1
  cyemi_825/1 -> cfblk37/1
  cyemi_826/1 -> cfblk38/1
  cfblk69/1 -> cyemi_826/1
  cyemi_827/1 -> cfblk38/2
  cfblk11/1 -> cyemi_827/1
  cyemi_828/1 -> cfblk39/1
  cfblk204/1(cfblk2) -> cyemi_828/1
  cyemi_829/1 -> cfblk4/1
  cfblk198/1(cfblk2) -> cyemi_829/1
  cyemi_830/1 -> cfblk40/1
  cfblk85/1 -> cyemi_830/1
  cyemi_831/1 -> cfblk41/1
  cfblk201/3(cfblk12) -> cyemi_831/1
  cyemi_832/1 -> cfblk42/1
  cfblk221/1 -> cyemi_832/1
  cyemi_833/1 -> cfblk42/2
  cfblk190/2(cfblk14) -> cyemi_833/1
  cyemi_834/1 -> cfblk43/1
  cfblk147/1 -> cyemi_834/1
  cyemi_835/1 -> cfblk44/1
  cfblk189/1(cfblk2) -> cyemi_835/1
  cyemi_836/1 -> cfblk45/1
  cfblk58/1 -> cyemi_836/1
  cyemi_837/1 -> cfblk46/1
  cfblk25/1 -> cyemi_837/1
  cyemi_838/1 -> cfblk47/1
  cyemi_839/1 -> cfblk47/2
  cyemi_840/1 -> cfblk48/1
  cfblk197/4(cfblk17) -> cyemi_840/1
  cyemi_841/1 -> cfblk49/1
  cfblk187/2(cfblk16) -> cyemi_841/1
  cyemi_842/1 -> cfblk5/1
  cfblk199/1(cfblk2) -> cyemi_842/1
  cyemi_843/1 -> cfblk50/1
  cyemi_844/1 -> cfblk51/1
  cfblk55/1 -> cyemi_844/1
  cyemi_845/1 -> cfblk52/1
  cfblk195/1(cfblk2) -> cyemi_845/1
  cyemi_846/1 -> cfblk53/1
  cyemi_847/1 -> cfblk54/1
  cfblk67/1 -> cyemi_847/1
  cyemi_848/1 -> cfblk55/1
  cfblk159/1 -> cyemi_848/1
  cyemi_849/1 -> cfblk56/1
  cfblk204/2(cfblk9) -> cyemi_849/1
  cyemi_850/1 -> cfblk57/1
  cfblk136/1 -> cyemi_850/1
  cyemi_851/1 -> cfblk57/2
  cfblk29/1 -> cyemi_851/1
  cyemi_852/1 -> cfblk58/1
  cfblk40/1 -> cyemi_852/1
  cyemi_853/1 -> cfblk59/1
  cfblk140/1 -> cyemi_853/1
  cyemi_854/1 -> cfblk6/1
  cfblk143/1 -> cyemi_854/1
  cyemi_855/1 -> cfblk60/1
  cfblk213/1 -> cyemi_855/1
  cyemi_856/1 -> cfblk60/2
  cfblk78/1 -> cyemi_856/1
  cyemi_857/1 -> cfblk61/1
  cfblk192/1(cfblk2) -> cyemi_857/1
  cyemi_858/1 -> cfblk62/1
  cyemi_859/1 -> cfblk63/1
  cfblk207/1(cfblk2) -> cyemi_859/1
  cyemi_860/1 -> cfblk64/1
  cfblk196/1(cfblk2) -> cyemi_860/1
  cyemi_861/1 -> cfblk65/1
  cfblk201/4(cfblk13) -> cyemi_861/1
  cyemi_862/1 -> cfblk65/2
  cyemi_863/1 -> cfblk66/1
  cfblk166/1 -> cyemi_863/1
  cyemi_864/1 -> cfblk67/1
  cyemi_865/1 -> cfblk68/1
  cfblk79/1 -> cyemi_865/1
  cyemi_866/1 -> cfblk69/1
  cyemi_867/1 -> cfblk69/2
  cfblk190/3(cfblk15) -> cyemi_867/1
  cyemi_868/1 -> cfblk7/1
  cyemi_869/1 -> cfblk70/1
  cfblk139/1 -> cyemi_869/1
  cyemi_870/1 -> cfblk71/1
  cfblk169/1 -> cyemi_870/1
  cyemi_871/1 -> cfblk72/1
  cyemi_872/1 -> cfblk73/1
  cfblk187/1(cfblk2) -> cyemi_872/1
  cyemi_873/1 -> cfblk74/1
  cyemi_874/1 -> cfblk75/1
  cyemi_875/1 -> cfblk75/2
  cfblk163/1 -> cyemi_875/1
  cyemi_876/1 -> cfblk76/1
  cfblk83/1 -> cyemi_876/1
  cyemi_877/1 -> cfblk77/1
  cfblk7/1 -> cyemi_877/1
  cyemi_878/1 -> cfblk77/2
  cyemi_879/1 -> cfblk78/1
  cfblk57/1 -> cyemi_879/1
  cyemi_880/1 -> cfblk79/1
  cfblk35/1 -> cyemi_880/1
  cyemi_881/1 -> cfblk8/1
  cfblk209/2(cfblk14) -> cyemi_881/1
  cyemi_882/1 -> cfblk80/1
  cfblk145/1 -> cyemi_882/1
  cyemi_883/1 -> cfblk81/1
  cfblk194/1(cfblk2) -> cyemi_883/1
  cyemi_884/1 -> cfblk82/1
  cfblk81/1 -> cyemi_884/1
  cyemi_885/1 -> cfblk83/1
  cyemi_886/1 -> cfblk83/2
  cyemi_887/1 -> cfblk84/1
  cyemi_888/1 -> cfblk84/2
  cyemi_889/1 -> cfblk85/1
  cyemi_890/1 -> cfblk86/1
  cfblk33/1 -> cyemi_890/1
  cyemi_891/1 -> cfblk87/1
  cfblk157/1 -> cyemi_891/1
  cyemi_892/1 -> cfblk9/1
  cfblk195/3(cfblk16) -> cyemi_892/1
  cyemi_893/1 -> cfblk93/1

== system sampleModel7127_pp_difftest/cfblk162 ==
  Demux : Demux  Tag=STV Demux  Outputs=1
  FromWs : FromWorkspace  Tag=STV FromWs  VariableName=tuvar  SampleTime=0
      SigBuilderData=|
      | common.afterFinalStr = 'Extrapolate'
      | common.sampleTime = 0
      | dataSet.timeRange = [0 10]
      | dataSet.name = 'Group 1'
      | sbobj.Groups.Name = 'Group 1'
      | sbobj.Groups.Signals.Name = 'Signal 1'
      | sbobj.Groups.Signals.XData = [0 4 4 6 6 10]
      | sbobj.Groups.Signals.YData = [0 0 1 1 0 0]
  Signal 1 : Outport  Tag=STV Outport
  wires:
  Demux/1 -> Signal 1/1
  FromWs/1 -> Demux/1

== system sampleModel7127_pp_difftest/cfblk164 ==
  Demux : Demux  Tag=STV Demux  Outputs=1
  FromWs : FromWorkspace  Tag=STV FromWs  VariableName=tuvar  SampleTime=0
      SigBuilderData=|
      | common.afterFinalStr = 'Extrapolate'
      | common.sampleTime = 0
      | dataSet.timeRange = [0 10]
      | dataSet.name = 'Group 1'
      | sbobj.Groups.Name = 'Group 1'
      | sbobj.Groups.Signals.Name = 'Signal 1'
      | sbobj.Groups.Signals.XData = [0 4 4 6 6 10]
      | sbobj.Groups.Signals.YData = [0 0 1 1 0 0]
  Signal 1 : Outport  Tag=STV Outport
  wires:
  Demux/1 -> Signal 1/1
  FromWs/1 -> Demux/1

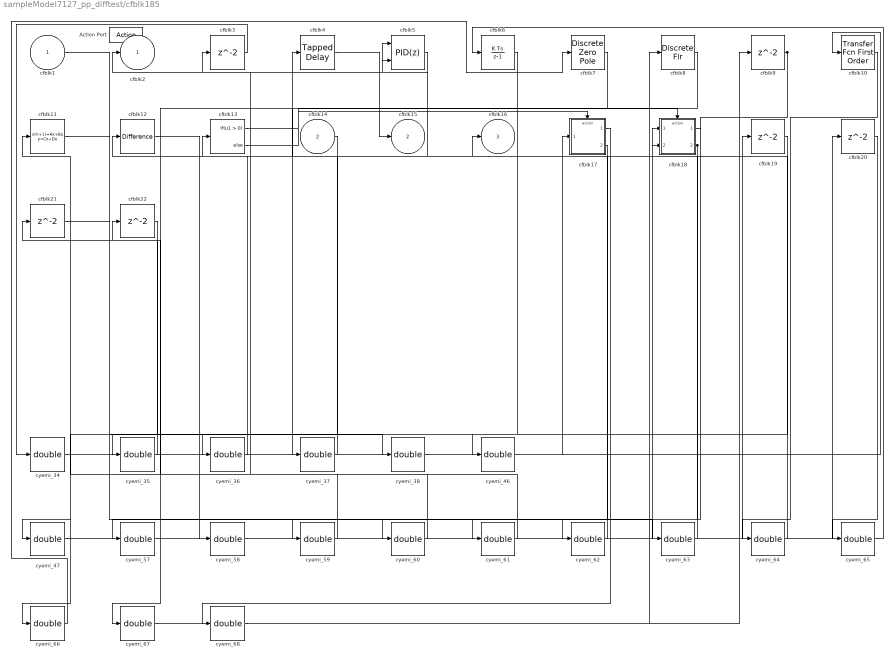
== system sampleModel7127_pp_difftest/cfblk185 ==
  cfblk1 : Inport
  cfblk14 : Inport  Port=2
  Action Port : ActionPort  ActionType=then
  cfblk10 : simulink/Discrete/Transfer Fcn First Order  PoleZ=0.95  ICPrevOutput=0.0  DoSatur=off
      settings: SourceProductName=Simulink
  cfblk11 : DiscreteStateSpace  SampleTime=-1
  cfblk12 : simulink/Discrete/Difference  ICPrevInput=0.0  OutMin=[]  OutMax=[]  OutDataTypeStr=double  OutputDataTypeScalingMode=double  OutDataType=fixdt(1, 16)  OutScaling=2^-10  DoSatur=off
  cfblk13 : If  SampleTime=1
  cfblk17 : Subsystem  TreatAsAtomicUnit=on
  cfblk18 : Subsystem  TreatAsAtomicUnit=on
  cfblk{3,9,19..22} (6 alike) : Delay
  cfblk4 : simulink/Discrete/Tapped Delay  vinit=0.0  samptime=-1  NumDelays=1  DelayOrder=Oldest  includeCurrent=off
  cfblk5 : simulink/Continuous/PID Controller (2DOF)  Controller=PID  TimeDomain=Discrete-time  SampleTime=-1  IntegratorMethod=Forward Euler  FilterMethod=Forward Euler  Form=Parallel  UseFilter=on  ControllerParametersSource=internal  P=1  I=1  D=0  N=100  b=1  c=1  InitialConditionSource=internal  InitialConditionForIntegrator=0  InitialConditionForFilter=0  ExternalReset=none  LimitOutput=off  UpperSaturationLimit=inf  LowerSaturationLimit=-inf  LinearizeAsGain=off  AntiWindupMode=none  Kb=1  TrackingMode=off  Kt=1  PParamMin=[]  PParamMax=[]  IParamMin=[]  IParamMax=[]  DParamMin=[]  DParamMax=[]  NParamMin=[]  NParamMax=[]  bParamMin=[]  bParamMax=[]  cParamMin=[]  cParamMax=[]  KbParamMin=[]  KbParamMax=[]  KtParamMin=[]  KtParamMax=[]  POutMin=[]  POutMax=[]  IOutMin=[]  IOutMax=[]  DOutMin=[]  DOutMax=[]  NOutMin=[]  NOutMax=[]  bOutMin=[]  bOutMax=[]  cOutMin=[]  cOutMax=[]  KbOutMin=[]  KbOutMax=[]  KtOutMin=[]  KtOutMax=[]  IntegratorOutMin=[]  IntegratorOutMax=[]  FilterOutMin=[]  FilterOutMax=[]  SumOutMin=[]  SumOutMax=[]  Sum1OutMin=[]  Sum1OutMax=[]  Sum2OutMin=[]  Sum2OutMax=[]  Sum3OutMin=[]  Sum3OutMax=[]  SumI1OutMin=[]  SumI1OutMax=[]  SumI2OutMin=[]  SumI2OutMax=[]  SumI3OutMin=[]  SumI3OutMax=[]  SumDOutMin=[]  SumDOutMax=[]  SaturationOutMin=[]  SaturationOutMax=[]  IntegratorContinuousStateAttributes=''  IntegratorStateMustResolveToSignalObject=off  IntegratorRTWStateStorageClass=Auto  FilterContinuousStateAttributes=''  FilterStateMustResolveToSignalObject=off  FilterRTWStateStorageClass=Auto  DifferentiatorICPrevScaledInput=0  DifferentiatorOutMin=[]  DifferentiatorOutMax=[]  FilterDiffOutCoefMin=[]  FilterDiffOutCoefMax=[]  SumDenOutMin=[]  SumDenOutMax=[]  SumNumOutMin=[]  SumNumOutMax=[]  ReciprocalOutMin=[]  ReciprocalOutMax=[]  DivideOutMin=[]  DivideOutMax=[]  TunerSelectOption=Transfer Function Based (PID Tuner App)
  cfblk6 : DiscreteIntegrator  SampleTime=-1  OutDataTypeStr=double  ICPrevOutput=DiscIntNeverNeededParam  ICPrevScaledInput=DiscIntNeverNeededParam
  cfblk7 : DiscreteZeroPole  Poles=[0 0.5]  Gain=1  SampleTime=-1
  cfblk8 : DiscreteFir
  cyemi_{34..38,46..47,57..68} (19 alike) : DataTypeConversion  OutDataTypeStr=double
  cfblk2 : Outport
  cfblk15 : Outport  Port=2
  cfblk16 : Outport  Port=3
  wires:
  cfblk5/1 -> cfblk2/1
  cfblk4/1 -> cfblk15/1
  cfblk9/1 -> cyemi_57/1, cyemi_60/1
  cfblk18/2(cfblk10) -> cfblk16/1, cyemi_59/1
  cfblk13/1 -> cfblk17/Action
  cfblk13/2 -> cfblk18/Action
  cyemi_34/1 -> cfblk10/1
  cfblk3/1 -> cyemi_34/1
  cyemi_35/1 -> cfblk11/1
  cfblk7/1 -> cyemi_35/1
  cyemi_36/1 -> cfblk12/1
  cfblk18/1(cfblk2) -> cyemi_36/1
  cyemi_37/1 -> cfblk13/1
  cfblk8/1 -> cyemi_37/1
  cyemi_38/1 -> cfblk17/1(cfblk1)
  cfblk21/1 -> cyemi_38/1
  cyemi_46/1 -> cfblk18/1(cfblk1)
  cfblk19/1 -> cyemi_46/1
  cyemi_47/1 -> cfblk18/2(cfblk9)
  cfblk22/1 -> cyemi_47/1
  cyemi_57/1 -> cfblk19/1
  cyemi_58/1 -> cfblk20/1
  cfblk12/1 -> cyemi_58/1
  cyemi_59/1 -> cfblk21/1
  cyemi_60/1 -> cfblk22/1
  cyemi_61/1 -> cfblk3/1
  cfblk11/1 -> cyemi_61/1
  cyemi_62/1 -> cfblk4/1
  cfblk17/2(cfblk8) -> cyemi_62/1
  cyemi_63/1 -> cfblk5/1
  cfblk1/1 -> cyemi_63/1
  cyemi_64/1 -> cfblk5/2
  cfblk10/1 -> cyemi_64/1
  cyemi_65/1 -> cfblk6/1
  cfblk20/1 -> cyemi_65/1
  cyemi_66/1 -> cfblk7/1
  cfblk14/1 -> cyemi_66/1
  cyemi_67/1 -> cfblk8/1
  cfblk6/1 -> cyemi_67/1
  cyemi_68/1 -> cfblk9/1
  cfblk17/1(cfblk2) -> cyemi_68/1

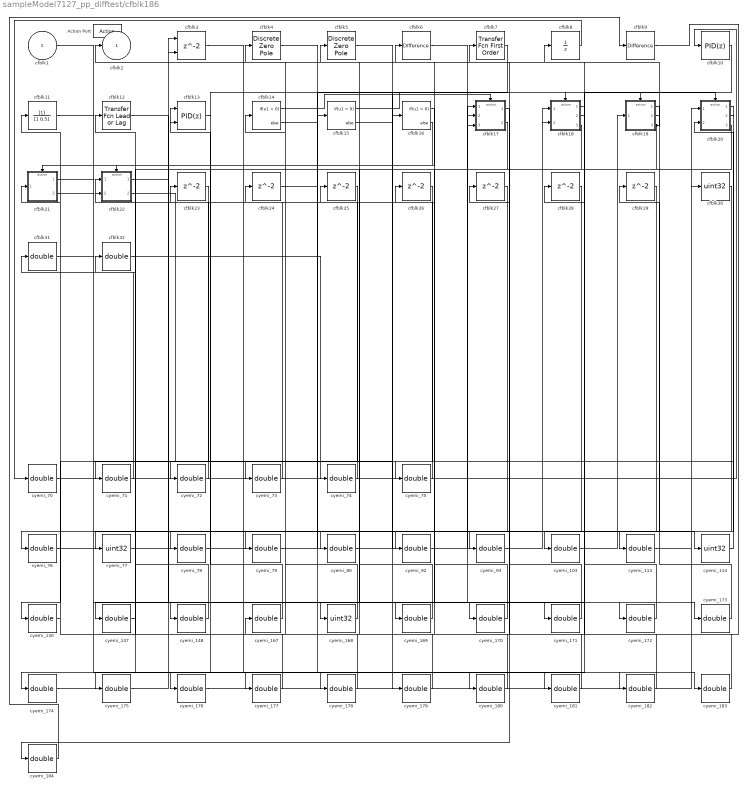
== system sampleModel7127_pp_difftest/cfblk186 ==
  cfblk1 : Inport
  Action Port : ActionPort  ActionType=else
  cfblk10 : simulink/Continuous/PID Controller  Controller=PID  TimeDomain=Discrete-time  SampleTime=-1  IntegratorMethod=Forward Euler  FilterMethod=Forward Euler  Form=Parallel  UseFilter=on  ControllerParametersSource=internal  P=1  I=1  D=0  N=100  InitialConditionSource=internal  InitialConditionForIntegrator=0  InitialConditionForFilter=0  ExternalReset=none  LimitOutput=off  UpperSaturationLimit=inf  LowerSaturationLimit=-inf  LinearizeAsGain=off  AntiWindupMode=none  Kb=1  TrackingMode=off  Kt=1  PParamMin=[]  PParamMax=[]  IParamMin=[]  IParamMax=[]  DParamMin=[]  DParamMax=[]  NParamMin=[]  NParamMax=[]  KbParamMin=[]  KbParamMax=[]  KtParamMin=[]  KtParamMax=[]  POutMin=[]  POutMax=[]  IOutMin=[]  IOutMax=[]  DOutMin=[]  DOutMax=[]  NOutMin=[]  NOutMax=[]  KbOutMin=[]  KbOutMax=[]  KtOutMin=[]  KtOutMax=[]  IntegratorOutMin=[]  IntegratorOutMax=[]  FilterOutMin=[]  FilterOutMax=[]  SumOutMin=[]  SumOutMax=[]  SumI1OutMin=[]  SumI1OutMax=[]  SumI2OutMin=[]  SumI2OutMax=[]  SumI3OutMin=[]  SumI3OutMax=[]  SumDOutMin=[]  SumDOutMax=[]  SaturationOutMin=[]  SaturationOutMax=[]  IntegratorContinuousStateAttributes=''  IntegratorStateMustResolveToSignalObject=off  IntegratorRTWStateStorageClass=Auto  FilterContinuousStateAttributes=''  FilterStateMustResolveToSignalObject=off  FilterRTWStateStorageClass=Auto  DifferentiatorICPrevScaledInput=0  DifferentiatorOutMin=[]  DifferentiatorOutMax=[]  FilterDiffOutCoefMin=[]  FilterDiffOutCoefMax=[]  SumDenOutMin=[]  SumDenOutMax=[]  SumNumOutMin=[]  SumNumOutMax=[]  ReciprocalOutMin=[]  ReciprocalOutMax=[]  DivideOutMin=[]  DivideOutMax=[]  TunerSelectOption=Transfer Function Based (PID Tuner App)
  cfblk11 : DiscreteFilter
  cfblk12 : simulink/Discrete/Transfer Fcn Lead or Lag  PoleZ=0.95  ZeroZ=0.75  ICPrevOutput=0.0  ICPrevInput=0.0  DoSatur=off
      settings: SourceProductName=Simulink  SourceProductBaseCode=SL
  cfblk13 : simulink/Continuous/PID Controller (2DOF)  Controller=PID  TimeDomain=Discrete-time  SampleTime=-1  IntegratorMethod=Forward Euler  FilterMethod=Forward Euler  Form=Parallel  UseFilter=on  ControllerParametersSource=internal  P=1  I=1  D=0  N=100  b=1  c=1  InitialConditionSource=internal  InitialConditionForIntegrator=0  InitialConditionForFilter=0  ExternalReset=none  LimitOutput=off  UpperSaturationLimit=inf  LowerSaturationLimit=-inf  LinearizeAsGain=off  AntiWindupMode=none  Kb=1  TrackingMode=off  Kt=1  PParamMin=[]  PParamMax=[]  IParamMin=[]  IParamMax=[]  DParamMin=[]  DParamMax=[]  NParamMin=[]  NParamMax=[]  bParamMin=[]  bParamMax=[]  cParamMin=[]  cParamMax=[]  KbParamMin=[]  KbParamMax=[]  KtParamMin=[]  KtParamMax=[]  POutMin=[]  POutMax=[]  IOutMin=[]  IOutMax=[]  DOutMin=[]  DOutMax=[]  NOutMin=[]  NOutMax=[]  bOutMin=[]  bOutMax=[]  cOutMin=[]  cOutMax=[]  KbOutMin=[]  KbOutMax=[]  KtOutMin=[]  KtOutMax=[]  IntegratorOutMin=[]  IntegratorOutMax=[]  FilterOutMin=[]  FilterOutMax=[]  SumOutMin=[]  SumOutMax=[]  Sum1OutMin=[]  Sum1OutMax=[]  Sum2OutMin=[]  Sum2OutMax=[]  Sum3OutMin=[]  Sum3OutMax=[]  SumI1OutMin=[]  SumI1OutMax=[]  SumI2OutMin=[]  SumI2OutMax=[]  SumI3OutMin=[]  SumI3OutMax=[]  SumDOutMin=[]  SumDOutMax=[]  SaturationOutMin=[]  SaturationOutMax=[]  IntegratorContinuousStateAttributes=''  IntegratorStateMustResolveToSignalObject=off  IntegratorRTWStateStorageClass=Auto  FilterContinuousStateAttributes=''  FilterStateMustResolveToSignalObject=off  FilterRTWStateStorageClass=Auto  DifferentiatorICPrevScaledInput=0  DifferentiatorOutMin=[]  DifferentiatorOutMax=[]  FilterDiffOutCoefMin=[]  FilterDiffOutCoefMax=[]  SumDenOutMin=[]  SumDenOutMax=[]  SumNumOutMin=[]  SumNumOutMax=[]  ReciprocalOutMin=[]  ReciprocalOutMax=[]  DivideOutMin=[]  DivideOutMax=[]  TunerSelectOption=Transfer Function Based (PID Tuner App)
  cfblk14 : If  SampleTime=1
  cfblk15 : If  SampleTime=1
  cfblk16 : If  SampleTime=1
  cfblk17 : Subsystem  TreatAsAtomicUnit=on
  cfblk18 : Subsystem  TreatAsAtomicUnit=on
  cfblk19 : Subsystem  TreatAsAtomicUnit=on
  cfblk20 : Subsystem  TreatAsAtomicUnit=on
  cfblk21 : Subsystem  TreatAsAtomicUnit=on
  cfblk22 : Subsystem  TreatAsAtomicUnit=on
  cfblk{23..29} (7 alike) : Delay
  cfblk3 : Delay  ShowEnablePort=on
      settings: InputPortMap=u0,e6
  cfblk30 : DataTypeConversion  OutDataTypeStr=uint32
  cfblk31 : DataTypeConversion  OutDataTypeStr=double
  cfblk32 : DataTypeConversion  OutDataTypeStr=double
  cfblk4 : DiscreteZeroPole  Poles=[0 0.5]  Gain=1  SampleTime=-1
  cfblk5 : DiscreteZeroPole  Poles=[0 0.5]  Gain=1  SampleTime=-1
  cfblk6 : simulink/Discrete/Difference  ICPrevInput=0.0  OutMin=[]  OutMax=[]  OutDataTypeStr=double  OutputDataTypeScalingMode=double  OutDataType=fixdt(1, 16)  OutScaling=2^-10  DoSatur=off
  cfblk7 : simulink/Discrete/Transfer Fcn First Order  PoleZ=0.95  ICPrevOutput=0.0  DoSatur=off
      settings: SourceProductName=Simulink
  cfblk8 : UnitDelay  SampleTime=-1
  cfblk9 : simulink/Discrete/Difference  ICPrevInput=0.0  OutMin=[]  OutMax=[]  OutDataTypeStr=double  OutputDataTypeScalingMode=double  OutDataType=fixdt(1, 16)  OutScaling=2^-10  DoSatur=off
  cyemi_{70..76,78..80,92..93,103,113,130,147..148,167,169..184} (34 alike) : DataTypeConversion  OutDataTypeStr=double
  cyemi_114 : DataTypeConversion  OutDataTypeStr=uint32
  cyemi_168 : DataTypeConversion  OutDataTypeStr=uint32
  cyemi_77 : DataTypeConversion  OutDataTypeStr=uint32
  cfblk2 : Outport
  wires:
  cfblk19/3(cfblk11) -> cfblk2/1, cyemi_80/1
  cfblk14/1 -> cfblk17/Action
  cfblk14/2 -> cfblk18/Action
  cfblk15/1 -> cfblk19/Action
  cfblk15/2 -> cfblk20/Action
  cfblk16/1 -> cfblk21/Action
  cfblk16/2 -> cfblk22/Action
  cyemi_70/1 -> cfblk10/1
  cfblk8/1 -> cyemi_70/1
  cyemi_71/1 -> cfblk11/1
  cfblk20/2(cfblk15) -> cyemi_71/1
  cyemi_72/1 -> cfblk12/1
  cfblk7/1 -> cyemi_72/1
  cyemi_73/1 -> cfblk13/1
  cfblk31/1 -> cyemi_73/1
  cyemi_74/1 -> cfblk13/2
  cfblk32/1 -> cyemi_74/1
  cyemi_75/1 -> cfblk14/1
  cfblk26/1 -> cyemi_75/1
  cyemi_76/1 -> cfblk15/1
  cfblk29/1 -> cyemi_76/1
  cyemi_77/1 -> cfblk16/1
  cfblk20/3(cfblk16) -> cyemi_77/1
  cyemi_78/1 -> cfblk17/1(cfblk1)
  cfblk28/1 -> cyemi_78/1
  cyemi_79/1 -> cfblk17/2(cfblk13)
  cfblk19/2(cfblk10) -> cyemi_79/1
  cyemi_80/1 -> cfblk17/3(cfblk14)
  cyemi_92/1 -> cfblk18/1(cfblk1)
  cfblk19/1(cfblk2) -> cyemi_92/1
  cyemi_93/1 -> cfblk18/2(cfblk9)
  cfblk27/1 -> cyemi_93/1
  cyemi_103/1 -> cfblk19/1(cfblk1)
  cfblk20/1(cfblk2) -> cyemi_103/1
  cyemi_113/1 -> cfblk20/1(cfblk1)
  cfblk1/1 -> cyemi_113/1
  cyemi_114/1 -> cfblk20/2(cfblk14)
  cfblk24/1 -> cyemi_114/1
  cyemi_130/1 -> cfblk21/1(cfblk1)
  cfblk23/1 -> cyemi_130/1
  cyemi_147/1 -> cfblk22/1(cfblk1)
  cfblk18/1(cfblk2) -> cyemi_147/1
  cyemi_148/1 -> cfblk22/2(cfblk15)
  cfblk25/1 -> cyemi_148/1
  cyemi_167/1 -> cfblk23/1
  cfblk9/1 -> cyemi_167/1
  cyemi_168/1 -> cfblk24/1
  cfblk30/1 -> cyemi_168/1
  cyemi_169/1 -> cfblk25/1
  cfblk17/2(cfblk15) -> cyemi_169/1
  cyemi_170/1 -> cfblk26/1
  cfblk22/1(cfblk2) -> cyemi_170/1
  cyemi_171/1 -> cfblk27/1
  cfblk12/1 -> cyemi_171/1
  cyemi_172/1 -> cfblk28/1
  cfblk6/1 -> cyemi_172/1
  cyemi_173/1 -> cfblk29/1
  cfblk11/1 -> cyemi_173/1
  cyemi_174/1 -> cfblk3/1
  cfblk18/2(cfblk10) -> cyemi_174/1
  cyemi_175/1 -> cfblk3/2
  cfblk18/3(cfblk11) -> cyemi_175/1
  cyemi_176/1 -> cfblk30/1
  cfblk13/1 -> cyemi_176/1
  cyemi_177/1 -> cfblk31/1
  cfblk21/1(cfblk2) -> cyemi_177/1
  cyemi_178/1 -> cfblk32/1
  cfblk21/2(cfblk16) -> cyemi_178/1
  cyemi_179/1 -> cfblk4/1
  cfblk22/2(cfblk16) -> cyemi_179/1
  cyemi_180/1 -> cfblk5/1
  cfblk4/1 -> cyemi_180/1
  cyemi_181/1 -> cfblk6/1
  cfblk10/1 -> cyemi_181/1
  cyemi_182/1 -> cfblk7/1
  cfblk5/1 -> cyemi_182/1
  cyemi_183/1 -> cfblk8/1
  cfblk3/1 -> cyemi_183/1
  cyemi_184/1 -> cfblk9/1
  cfblk17/1(cfblk2) -> cyemi_184/1

== system sampleModel7127_pp_difftest/cfblk187 ==
  cfblk1 : Inport
  cfblk13 : Inport  Port=2
  cfblk14 : Inport  Port=3
  cfblk15 : Inport  Port=4
  Action Port : ActionPort  ActionType=then
  cfblk10 : simulink/Discrete/Tapped Delay  vinit=0.0  samptime=-1  NumDelays=1  DelayOrder=Oldest  includeCurrent=off
  cfblk11 : DiscreteStateSpace  SampleTime=-1
  cfblk12 : UnitDelay  SampleTime=-1
  cfblk17 : DataTypeConversion  OutDataTypeStr=uint32
  cfblk18 : DataTypeConversion  OutDataTypeStr=double
  cfblk19 : DataTypeConversion  OutDataTypeStr=double
  cfblk20 : DataTypeConversion  OutDataTypeStr=double
  cfblk3 : Delay  DelayLengthSource=Input port
      settings: InputPortMap=u0,p1
  cfblk4 : simulink/Continuous/PID Controller  Controller=PID  TimeDomain=Discrete-time  SampleTime=-1  IntegratorMethod=Forward Euler  FilterMethod=Forward Euler  Form=Parallel  UseFilter=on  ControllerParametersSource=internal  P=1  I=1  D=0  N=100  InitialConditionSource=internal  InitialConditionForIntegrator=0  InitialConditionForFilter=0  ExternalReset=none  LimitOutput=off  UpperSaturationLimit=inf  LowerSaturationLimit=-inf  LinearizeAsGain=off  AntiWindupMode=none  Kb=1  TrackingMode=off  Kt=1  PParamMin=[]  PParamMax=[]  IParamMin=[]  IParamMax=[]  DParamMin=[]  DParamMax=[]  NParamMin=[]  NParamMax=[]  KbParamMin=[]  KbParamMax=[]  KtParamMin=[]  KtParamMax=[]  POutMin=[]  POutMax=[]  IOutMin=[]  IOutMax=[]  DOutMin=[]  DOutMax=[]  NOutMin=[]  NOutMax=[]  KbOutMin=[]  KbOutMax=[]  KtOutMin=[]  KtOutMax=[]  IntegratorOutMin=[]  IntegratorOutMax=[]  FilterOutMin=[]  FilterOutMax=[]  SumOutMin=[]  SumOutMax=[]  SumI1OutMin=[]  SumI1OutMax=[]  SumI2OutMin=[]  SumI2OutMax=[]  SumI3OutMin=[]  SumI3OutMax=[]  SumDOutMin=[]  SumDOutMax=[]  SaturationOutMin=[]  SaturationOutMax=[]  IntegratorContinuousStateAttributes=''  IntegratorStateMustResolveToSignalObject=off  IntegratorRTWStateStorageClass=Auto  FilterContinuousStateAttributes=''  FilterStateMustResolveToSignalObject=off  FilterRTWStateStorageClass=Auto  DifferentiatorICPrevScaledInput=0  DifferentiatorOutMin=[]  DifferentiatorOutMax=[]  FilterDiffOutCoefMin=[]  FilterDiffOutCoefMax=[]  SumDenOutMin=[]  SumDenOutMax=[]  SumNumOutMin=[]  SumNumOutMax=[]  ReciprocalOutMin=[]  ReciprocalOutMax=[]  DivideOutMin=[]  DivideOutMax=[]  TunerSelectOption=Transfer Function Based (PID Tuner App)
  cfblk5 : UnitDelay  SampleTime=-1
  cfblk6 : simulink/Discrete/Transfer Fcn Real Zero  ZeroZ=0.75  ICPrevInput=0.0  DoSatur=off
      settings: SourceProductName=Simulink  SourceProductBaseCode=SL
  cfblk7 : DiscreteFilter
  cfblk8 : simulink/Discrete/Transfer Fcn Lead or Lag  PoleZ=0.95  ZeroZ=0.75  ICPrevOutput=0.0  ICPrevInput=0.0  DoSatur=off
      settings: SourceProductName=Simulink  SourceProductBaseCode=SL
  cfblk9 : DiscreteFir
  cyemi_{189..194,196,198..203} (13 alike) : DataTypeConversion  OutDataTypeStr=double
  cyemi_195 : DataTypeConversion  OutDataTypeStr=fixdt('ufix64_En32')
  cyemi_197 : DataTypeConversion  OutDataTypeStr=uint32
  cfblk2 : Outport
  cfblk16 : Outport  Port=2
  wires:
  cfblk5/1 -> cfblk2/1
  cfblk13/1 -> cfblk16/1
  cyemi_189/1 -> cfblk10/1
  cfblk15/1 -> cyemi_189/1
  cyemi_190/1 -> cfblk11/1
  cfblk1/1 -> cyemi_190/1
  cyemi_191/1 -> cfblk12/1
  cfblk9/1 -> cyemi_191/1
  cyemi_192/1 -> cfblk17/1
  cfblk8/1 -> cyemi_192/1
  cyemi_193/1 -> cfblk18/1
  cfblk19/1 -> cyemi_193/1
  cyemi_194/1 -> cfblk19/1
  cfblk7/1 -> cyemi_194/1
  cyemi_195/1 -> cfblk20/1
  cfblk14/1 -> cyemi_195/1
  cyemi_196/1 -> cfblk3/1
  cfblk12/1 -> cyemi_196/1
  cyemi_197/1 -> cfblk3/2
  cfblk17/1 -> cyemi_197/1
  cyemi_198/1 -> cfblk4/1
  cfblk11/1 -> cyemi_198/1
  cyemi_199/1 -> cfblk5/1
  cfblk6/1 -> cyemi_199/1
  cyemi_200/1 -> cfblk6/1
  cfblk3/1 -> cyemi_200/1
  cyemi_201/1 -> cfblk7/1
  cfblk20/1 -> cyemi_201/1
  cyemi_202/1 -> cfblk8/1
  cfblk18/1 -> cyemi_202/1
  cyemi_203/1 -> cfblk9/1
  cfblk4/1 -> cyemi_203/1

== system sampleModel7127_pp_difftest/cfblk188 ==
  cfblk1 : Inport
  Action Port : ActionPort  ActionType=else
  cfblk10 : DiscreteTransferFcn
  cfblk3 : DiscreteFir
  cfblk4 : DiscreteTransferFcn
  cfblk5 : DiscreteIntegrator  SampleTime=-1  OutDataTypeStr=double  ICPrevOutput=DiscIntNeverNeededParam  ICPrevScaledInput=DiscIntNeverNeededParam
  cfblk6 : DiscreteFilter
  cfblk7 : DiscreteTransferFcn
  cfblk8 : simulink/Discrete/Transfer Fcn First Order  PoleZ=0.95  ICPrevOutput=0.0  DoSatur=off
      settings: SourceProductName=Simulink
  cfblk9 : simulink/Discrete/Tapped Delay  vinit=0.0  samptime=-1  NumDelays=1  DelayOrder=Oldest  includeCurrent=off
  cyemi_{205..212} (8 alike) : DataTypeConversion  OutDataTypeStr=double
  cfblk2 : Outport
  cfblk11 : Outport  Port=2
  wires:
  cfblk10/1 -> cfblk11/1
  cfblk5/1 -> cfblk2/1
  cfblk3/1 -> cyemi_205/1, cyemi_207/1
  cyemi_205/1 -> cfblk10/1
  cyemi_206/1 -> cfblk3/1
  cfblk9/1 -> cyemi_206/1
  cyemi_207/1 -> cfblk4/1
  cyemi_208/1 -> cfblk5/1
  cfblk8/1 -> cyemi_208/1
  cyemi_209/1 -> cfblk6/1
  cfblk7/1 -> cyemi_209/1
  cyemi_210/1 -> cfblk7/1
  cfblk4/1 -> cyemi_210/1
  cyemi_211/1 -> cfblk8/1
  cfblk6/1 -> cyemi_211/1
  cyemi_212/1 -> cfblk9/1
  cfblk1/1 -> cyemi_212/1

== system sampleModel7127_pp_difftest/cfblk189 ==
  cfblk1 : Inport
  cfblk7 : Inport  Port=2
  cfblk8 : Inport  Port=3
  Action Port : ActionPort  ActionType=then
  cfblk3 : Delay
  cfblk4 : simulink/Continuous/PID Controller  Controller=PID  TimeDomain=Discrete-time  SampleTime=-1  IntegratorMethod=Forward Euler  FilterMethod=Forward Euler  Form=Parallel  UseFilter=on  ControllerParametersSource=internal  P=1  I=1  D=0  N=100  InitialConditionSource=internal  InitialConditionForIntegrator=0  InitialConditionForFilter=0  ExternalReset=none  LimitOutput=off  UpperSaturationLimit=inf  LowerSaturationLimit=-inf  LinearizeAsGain=off  AntiWindupMode=none  Kb=1  TrackingMode=off  Kt=1  PParamMin=[]  PParamMax=[]  IParamMin=[]  IParamMax=[]  DParamMin=[]  DParamMax=[]  NParamMin=[]  NParamMax=[]  KbParamMin=[]  KbParamMax=[]  KtParamMin=[]  KtParamMax=[]  POutMin=[]  POutMax=[]  IOutMin=[]  IOutMax=[]  DOutMin=[]  DOutMax=[]  NOutMin=[]  NOutMax=[]  KbOutMin=[]  KbOutMax=[]  KtOutMin=[]  KtOutMax=[]  IntegratorOutMin=[]  IntegratorOutMax=[]  FilterOutMin=[]  FilterOutMax=[]  SumOutMin=[]  SumOutMax=[]  SumI1OutMin=[]  SumI1OutMax=[]  SumI2OutMin=[]  SumI2OutMax=[]  SumI3OutMin=[]  SumI3OutMax=[]  SumDOutMin=[]  SumDOutMax=[]  SaturationOutMin=[]  SaturationOutMax=[]  IntegratorContinuousStateAttributes=''  IntegratorStateMustResolveToSignalObject=off  IntegratorRTWStateStorageClass=Auto  FilterContinuousStateAttributes=''  FilterStateMustResolveToSignalObject=off  FilterRTWStateStorageClass=Auto  DifferentiatorICPrevScaledInput=0  DifferentiatorOutMin=[]  DifferentiatorOutMax=[]  FilterDiffOutCoefMin=[]  FilterDiffOutCoefMax=[]  SumDenOutMin=[]  SumDenOutMax=[]  SumNumOutMin=[]  SumNumOutMax=[]  ReciprocalOutMin=[]  ReciprocalOutMax=[]  DivideOutMin=[]  DivideOutMax=[]  TunerSelectOption=Transfer Function Based (PID Tuner App)
  cfblk5 : DiscreteStateSpace  SampleTime=-1
  cfblk6 : simulink/Discrete/Tapped Delay  vinit=0.0  samptime=-1  NumDelays=1  DelayOrder=Oldest  includeCurrent=off
  cyemi_{216..219} (4 alike) : DataTypeConversion  OutDataTypeStr=double
  cfblk2 : Outport
  wires:
  cfblk4/1 -> cfblk2/1
  cyemi_216/1 -> cfblk3/1
  cfblk7/1 -> cyemi_216/1
  cyemi_217/1 -> cfblk4/1
  cfblk3/1 -> cyemi_217/1
  cyemi_218/1 -> cfblk5/1
  cfblk8/1 -> cyemi_218/1
  cyemi_219/1 -> cfblk6/1
  cfblk5/1 -> cyemi_219/1
